simulink model "hinfinity"  (R2019b)
settings: Solver=VariableStepAuto  StartTime=0.0  StopTime=10.0  RelTol=1e-3
libraries: cstblocks x3
settings Model: Creator=Presentatie  LastModifiedBy=Presentatie

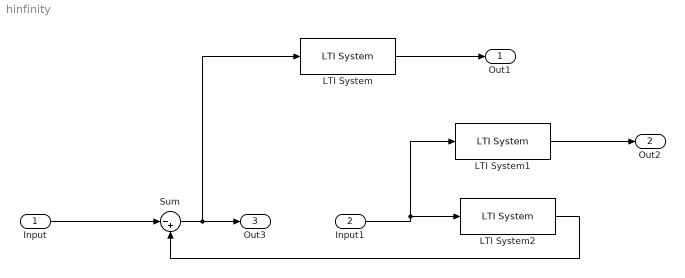
== system hinfinity ==
  Input : Inport
  Input1 : Inport  Port=2
  LTI System : cstblocks/LTI System  sys=Ws  IC=[]
  LTI System1 : cstblocks/LTI System  sys=Wu  IC=[]
  LTI System2 : cstblocks/LTI System  sys=G  IC=[]
  Sum : Sum  Inputs=|-+
  Out1 : Outport
  Out2 : Outport  Port=2
  Out3 : Outport  Port=3
  wires:
  Input1/1 -> LTI System2/1, LTI System1/1
  LTI System1/1 -> Out2/1
  Input/1 -> Sum/1
  Sum/1 -> Out3/1, LTI System/1
  LTI System2/1 -> Sum/2
  LTI System/1 -> Out1/1
